simulink model "processor"  (R2024a)
settings: Solver=VariableStepAuto  StartTime=0.0  StopTime=10.0  RelTol=1e-3
libraries: simulink x10, hdlsllib x6
settings Model: Creator=alehay  LastModifiedBy=alehay

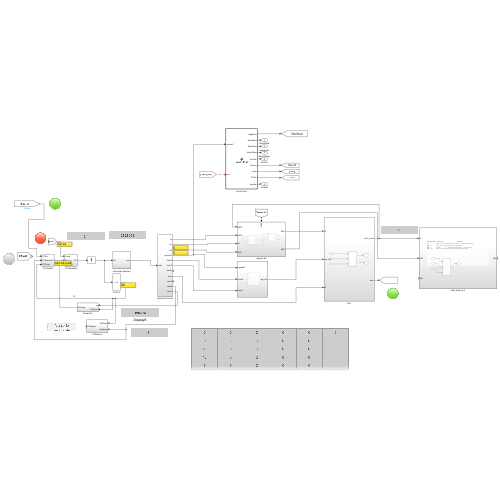
[thumbnail: Simulink's stored preview of the top-level diagram]
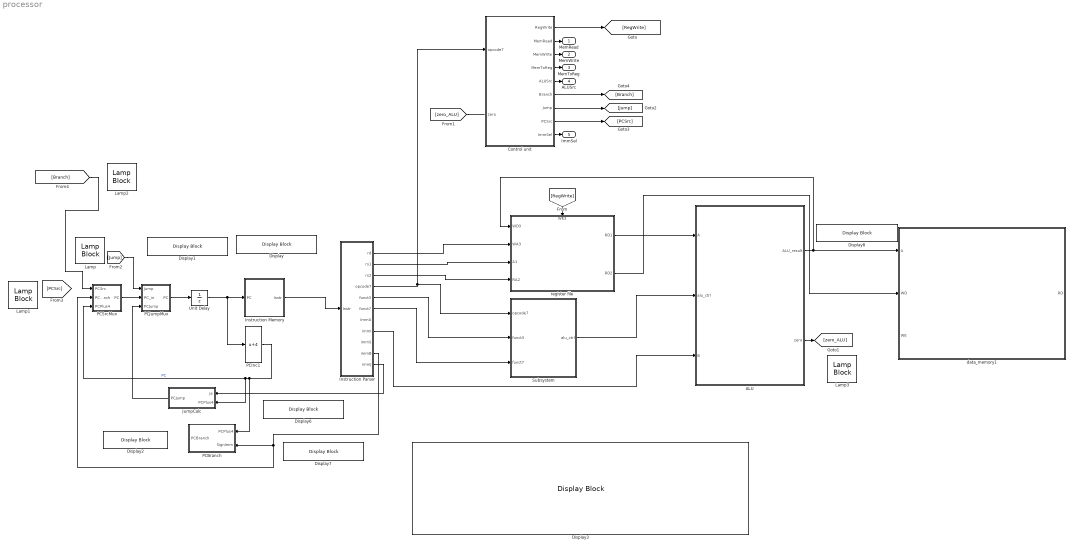
== system processor ==
  ALU : Subsystem
  Control unit : MATLAB Function  TreatAsAtomicUnit=on
  Display : DisplayBlock  LabelPosition=Hide  Format=Custom  Transparency=1  FormatString=%X
  Display{1,6..8} (4 alike) : DisplayBlock  LabelPosition=Hide  Transparency=1
  Display2 : DisplayBlock  LabelPosition=Hide  Format=long  Transparency=1
  Display3 : DisplayBlock  LabelPosition=Hide  Format=long  Transparency=1
  Instruction Memory : Subsystem
  Instruction Parser : Subsystem
  JumpCalc : Subsystem
  Lamp{,1..3} (4 alike) : LampBlock  LabelPosition=Hide
  PCBranch : Subsystem
  PCInc1 : Bias  Bias=4  SaturateOnIntegerOverflow=off
  PCJumpMux : Subsystem
  PCSrcMux : Subsystem
  Subsystem : Subsystem
  Unit Delay : UnitDelay  SampleTime=0.1  HasFrameUpgradeWarning=on
  data_memory1 : Subsystem
  register file : Subsystem
      settings: PortSchema="{\"entries\":[{\"content\":{\"sides\":[{\"content\":{\"connectorIds\":[\"In1\",\"In2\",\"In3\",\"In4\"]},\"type\":\"ConnectorPlacement.EquallySpacedRectSide\",\"uuid\":\"2ce0f731-262a-4c53-91f0-cda99c1614e4\"},{\"content\":{\"connectorIds\":[\"Out1\",\"Out2\"],\"side\":\"RIGHT\"},\"type\":\"ConnectorPlacement.EquallySpacedRectSide\",\"uuid\":\"7b2b7fe1-676c-4333-9af8-1b5ede950b35\"},{\"content\":{\"connectorIds\":[\"In5\"],\"side\":\"TOP\"},\"type\":\"ConnectorPlacement.EquallySpacedRectSide\",\"uuid\":\"79cd4f04-c8ad-45c4-b16c-19b290692dc4\"}]},\"type\":\"ConnectorPlacement.EquallySpacedConnector\",\"uuid\":\"48f070a2-9602-434c-b37d-35cc322e3ca0\"}],\"packageUris\":[\"http://schema.mathworks.com/mf0/Connector/R2020b\"],\"version\":\"1.0\"}"
  MemRead : Outport
  MemWrite : Outport  Port=2
  MemToReg : Outport  Port=3
  ALUSrc : Outport  Port=4
  ImmSel : Outport  Port=5
  wires:
  Control unit/5(ALUSrc) -> ALUSrc/1
  Instruction Parser/2(rs1) -> register file/3(A1)
  Control unit/9(ImmSel) -> ImmSel/1
  Control unit/3(MemWrite) -> MemWrite/1
  ALU/2(zero) -> [zero_ALU]
  Instruction Memory/1(Instr) -> Instruction Parser/1(Instr)
  Control unit/7(Jump) -> [Jump]
  register file/1(RD1) -> ALU/1(A)
  JumpCalc/1(PCJump) -> PCJumpMux/3(PCJump)
  register file/2(RD2) -> data_memory1/2(WD)
  Control unit/4(MemToReg) -> MemToReg/1
  Control unit/2(MemRead) -> MemRead/1
  Instruction Parser/6(funct7) -> Subsystem/3(funct7)
  Instruction Parser/4(opcode7) -> Control unit/1(opcode7), Subsystem/1(opcode7)
  [RegWrite] -> register file/5(WE3)
  Instruction Parser/5(funct3) -> Subsystem/2(funct3)
  PCInc1/1 -> PCSrcMux/3(PCPlus4), JumpCalc/2(PCPlus4), PCBranch/1(PCPlus4)  "PC"
  [zero_ALU] -> ?
  Control unit/1(RegWrite) -> [RegWrite]
  Instruction Parser/10(immB) -> PCSrcMux/2(PCBranch), PCBranch/2(SignImm)
  Instruction Parser/11(immJ) -> JumpCalc/1(ja)
  PCSrcMux/1(PC) -> PCJumpMux/2(PC_in)
  Control unit/8(PCSrc) -> [PCSrc]
  Unit Delay/1 -> Instruction Memory/1(PC), PCInc1/1
  Instruction Parser/3(rs2) -> register file/4(RA2)
  Control unit/6(Branch) -> [Branch]
  Instruction Parser/8(immI) -> ALU/3(B)
  Subsystem/1(alu_ctrl) -> ALU/2(alu_ctrl)
  [Jump] -> PCJumpMux/1(Jump)
  Instruction Parser/1(rd) -> register file/2(WA3)
  PCJumpMux/1(PC) -> Unit Delay/1
  ALU/1(ALU_result) -> data_memory1/1(A), register file/1(WD3)
  [Branch] -> PCSrcMux/1(PCSrc)

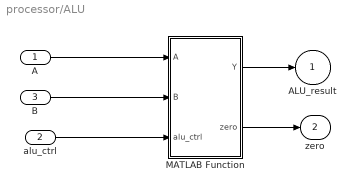
== system processor/ALU ==
  A : Inport
  alu_ctrl : Inport  Port=2
  B : Inport  Port=3
  MATLAB Function : MATLAB Function  TreatAsAtomicUnit=on
  ALU_result : Outport
  zero : Outport  Port=2
  wires:
  A/1 -> MATLAB Function/1(A)
  B/1 -> MATLAB Function/2(B)
  alu_ctrl/1 -> MATLAB Function/3(alu_ctrl)
  MATLAB Function/1(Y) -> ALU_result/1
  MATLAB Function/2(zero) -> zero/1

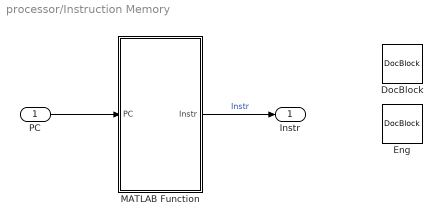
== system processor/Instruction Memory ==
  PC : Inport
  DocBlock : simulink/Model-Wide Utilities/DocBlock  DocumentType=Text
      content=|
      | Память команд имеет один порт чтения. На адресный вход A подается
      | 32-битный адрес команды, после чего на выходе RD появляется
      | 32-битное число (т.е. команда), прочитанное из памяти по этому адресу.
  Eng : simulink/Model-Wide Utilities/DocBlock  DocumentType=Text
      content=|
      | The instruction memory has a single read port.1 It takes a 32-bit
      | instruction address input, A, and reads the 32-bit data (i.e., instruction)
      | from that address onto the read data output, RD.
  MATLAB Function : MATLAB Function  TreatAsAtomicUnit=on
  Instr : Outport  OutDataTypeStr=fixdt(0,32,0)
  wires:
  PC/1 -> MATLAB Function/1(PC)
  MATLAB Function/1(Instr) -> Instr/1  "Instr"

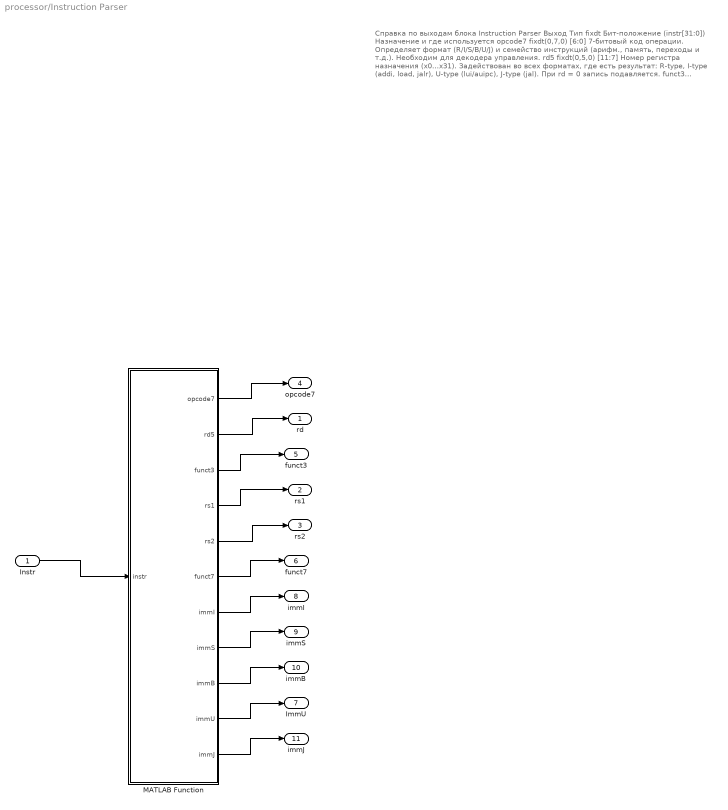
== system processor/Instruction Parser ==
  note: Справка по выходам блока Instruction Parser
      |
      | Выход
      | Тип fixdt
      | Бит-положение (instr[31:0])
      | Назначение и где используется
      |
      | opcode7
      | fixdt(0,7,0)
      | [6:0]
      | 7-битовый код операции. Определяет формат (R/I/S/B/U/J) и семейство инструкций (арифм., память, переходы и т.д.). Необходим для декодера управления.
      |
      | rd5
      | fixdt(0,5,0)
      | [11:7]
      | Номер регистра назначения (x0…x31). Задействован во всех форматах, где есть результат: R-type, I-type (addi, load, jalr), U-type (lui/auipc), J-type (jal). При rd = 0 запись подавляется.
      |
      | funct3
      | fixdt(0,3,0)
      | [14:12]
      | 3-битовое поле доп. кодировки операции. Совместно с opcode7 и/или funct7 окончательно выбирает инструкцию (например, add/sub, beq/bne/blt…).
      |
      | rs1
      | fixdt(0,5,0)
      | [19:15]
      | Номер первого исходного регистра. Используется во всех форматах, кроме U-type.
      |
      | rs2
      | fixdt(0,5,0)
      | [24:20]
      | Номер второго исходного регистра. Присутствует в R-type, S-type (store) и B-type (branch).
      |
      | funct7
      | fixdt(0,7,0)
      | [31:25]
      | 7-битовое поле расширенной функции. Отличает пары вроде add/sub, srl/sra, mul/div и др. Содержит 0x00, 0x20, 0x01 в базовом RV32IM.
      |
      | immI
      | fixdt(1,32,0)
      | sign-ext из [31:20]
      | 12-битное знаковое immed. для I-type (addi, lw, jalr, csrs …). Представляет диапазон −2048…+2047.
      |
      | immS
      | fixdt(1,32,0)
      | sign-ext из [31:25]+[11:7]
      | 12-битное знаковое immed. для S-type (store инструкции sw, sh, sb). Разделён на две части в коде.
      |
      | immB
      | fixdt(1,32,0)
      | sign-ext из [31], [7], [30:25], [11:8] затем <<1
      | 13-битное знаковое смещение для ветвлений B-type (beq, blt…). Младший бит всегда 0 — адрес выровнен по 2 байта. Диапазон ±4 кБ.
      |
      | immU
      | fixdt(1,32,0)
      | sign-ext из [31:12] затем <<12
      | 20-битное верхнее immediate для U-type (lui, auipc). Занимает старшие 20 бит результирующего слова, младшие 12 бит — нули.
      |
      | immJ
      | fixdt(1,32,0)
      | sign-ext из [31], [19:12], [20], [30:21]
      | 21-битное знаковое смещение для J-type (jal). Вычисляется с <<1; младший бит адреса всегда 0. Диапазон ±1 МБ.
  Instr : Inport
  MATLAB Function : MATLAB Function  TreatAsAtomicUnit=on
  rd : Outport
  rs1 : Outport  Port=2
  rs2 : Outport  Port=3
  opcode7 : Outport  Port=4
  funct3 : Outport  Port=5  OutDataTypeStr=fixdt(0,3,0)
  funct7 : Outport  Port=6  OutDataTypeStr=fixdt(0,7,0)
  ImmU : Outport  Port=7
  immI : Outport  Port=8
  immS : Outport  Port=9
  immB : Outport  Port=10
  immJ : Outport  Port=11
  wires:
  Instr/1 -> MATLAB Function/1(instr)
  MATLAB Function/1(opcode7) -> opcode7/1
  MATLAB Function/4(rs1) -> rs1/1
  MATLAB Function/3(funct3) -> funct3/1
  MATLAB Function/2(rd5) -> rd/1
  MATLAB Function/5(rs2) -> rs2/1
  MATLAB Function/6(funct7) -> funct7/1
  MATLAB Function/7(immI) -> immI/1
  MATLAB Function/8(immS) -> immS/1
  MATLAB Function/9(immB) -> immB/1
  MATLAB Function/10(immU) -> ImmU/1
  MATLAB Function/11(immJ) -> immJ/1

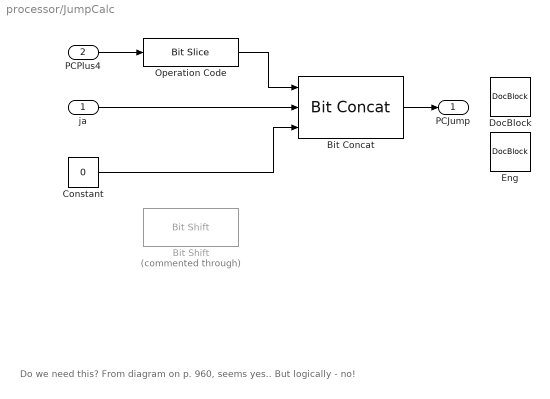
== system processor/JumpCalc ==
  note: Do we need this? From diagram on p. 960, seems yes.. But logically - no!
  ja : Inport
  PCPlus4 : Inport  Port=2
  Bit Concat : hdlsllib/Logic and Bit Operations/Bit Concat  numInputs=3
  Bit Shift : hdlsllib/Logic and Bit Operations/Bit Shift  Commented=through  mode=Shift Left Logical  N=2
  Constant : Constant  Value=0  OutDataTypeStr=fixdt(0,2,0)
  DocBlock : simulink/Model-Wide Utilities/DocBlock  DocumentType=Text
      content=|
      | Команда безусловного перехода j записывает новое значение в счетчик команд.
      | Два младших бита нового значения всегда равны нулю, потому что длина любой
      | команды равна четырем байтам, следовательно, ее адрес всегда кратен
      | четырем. Следующие 26 бит процессор возьмет из поля адреса перехода (jump
      | address field) Instr25:0. Четыре оставшихся старших бита будут равны четырем
      | старшим битам предыдущего значения счетчика команд.
  Eng : simulink/Model-Wide Utilities/DocBlock  DocumentType=Text
      content=|
      | The jump instruction, j, writes a new value into the PC. The two least significant
      | bits of the PC are always 0, because the PC is word aligned (i.e., always a multiple
      | of 4). The next 26 bits are taken from the jump address field in Instr25:0. The
      | upper four bits are taken from the old value of the PC.
  Operation Code : hdlsllib/Logic and Bit Operations/Bit Slice  lidx=31  ridx=28
  PCJump : Outport
  wires:
  Bit Concat/1 -> PCJump/1
  PCPlus4/1 -> Operation Code/1
  ja/1 -> Bit Concat/2
  Operation Code/1 -> Bit Concat/1
  Constant/1 -> Bit Concat/3

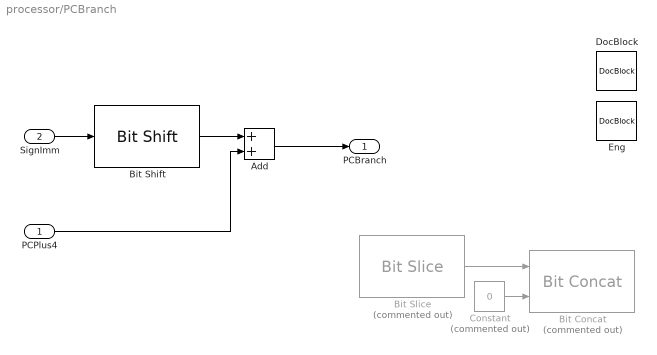
== system processor/PCBranch ==
  PCPlus4 : Inport
  SignImm : Inport  Port=2
  Add : Sum  OutDataTypeStr=fixdt(0,32,0)  AccumDataTypeStr=fixdt(0,32,0)
  Bit Concat : hdlsllib/Logic and Bit Operations/Bit Concat  Commented=on  numInputs=2
  Bit Shift : hdlsllib/Logic and Bit Operations/Bit Shift  mode=Shift Left Logical  N=2
  Bit Slice : hdlsllib/Logic and Bit Operations/Bit Slice  Commented=on  lidx=29  ridx=0
  Constant : Constant  Commented=on  Value=0  OutDataTypeStr=fixdt(0,2,0)
  DocBlock : simulink/Model-Wide Utilities/DocBlock  DocumentType=Text
      content=|
      | Смещение указывает, сколько команд нужно перепрыгнуть, прежде чем
      | продолжить выполнение программы. Таким образом, над значением
      | непосредственного операнда надо выполнить операцию знакового
      | расширения, поле чего умножить его на четыре, чтобы получить новое
      | значение счетчика команд: PC_in = PC + 4 + SignImm * 4.
      | Новое значение счетчика команд на случай выполненного
      | условного перехода (PCBranch) вычисляется путем сдвига SignImm
      | влево на два разряда и последующего сложения с PCPlus4.
  Eng : simulink/Model-Wide Utilities/DocBlock  DocumentType=Text
      content=|
      | The offset
      | indicates the number of instructions to branch past. Hence, the immediate
      | must be sign-extended and multiplied by 4 to get the new program counter
      | value: PC′ = PC + 4 + SignImm × 4.
      | The next PC value
      | for a taken branch, PCBranch, is computed by shifting SignImm left
      | by 2 bits, then adding it to PCPlus4.
  PCBranch : Outport
  wires:
  SignImm/1 -> Bit Shift/1
  PCPlus4/1 -> Add/2
  Bit Shift/1 -> Add/1
  Add/1 -> PCBranch/1
  Bit Slice/1 -> Bit Concat/1
  Constant/1 -> Bit Concat/2

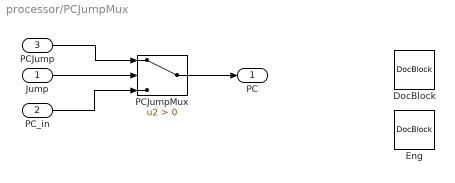
== system processor/PCJumpMux ==
  Jump : Inport
  PC_in : Inport  Port=2
  PCJump : Inport  Port=3
  DocBlock : simulink/Model-Wide Utilities/DocBlock  DocumentType=Text
      content=|
      | Команда безусловного перехода j записывает новое значение в счетчик команд.
      | Два младших бита нового значения всегда равны нулю, потому что длина любой
      | команды равна четырем байтам, следовательно, ее адрес всегда кратен
      | четырем. Следующие 26 бит процессор возьмет из поля адреса перехода (jump
      | address field) Instr25:0. Четыре оставшихся старших бита будут равны четырем
      | старшим битам предыдущего значения счетчика команд.
  Eng : simulink/Model-Wide Utilities/DocBlock  DocumentType=Text
      content=|
      | The jump instruction, j, writes a new value into the PC. The two least significant
      | bits of the PC are always 0, because the PC is word aligned (i.e., always a multiple
      | of 4). The next 26 bits are taken from the jump address field in Instr25:0. The
      | upper four bits are taken from the old value of the PC.
  PCJumpMux : Switch  Criteria=u2 > Threshold  SaturateOnIntegerOverflow=off  InputSameDT=off
  PC : Outport
  wires:
  PCJumpMux/1 -> PC/1
  Jump/1 -> PCJumpMux/2
  PCJump/1 -> PCJumpMux/1
  PC_in/1 -> PCJumpMux/3

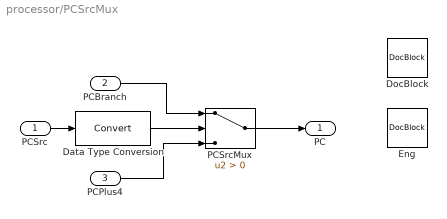
== system processor/PCSrcMux ==
  PCSrc : Inport  OutDataTypeStr=boolean
  PCBranch : Inport  Port=2
  PCPlus4 : Inport  Port=3
  Data Type Conversion : DataTypeConversion  SaturateOnIntegerOverflow=off  RndMeth=Floor
  DocBlock : simulink/Model-Wide Utilities/DocBlock  DocumentType=Text
      content=|
      | Мультиплексор, чтобы выбрать, какое именно
      | значение присвоить PC_in – PCPlus4 или PCBranch. PCBranch
      | используется тогда, когда выполняется команда условного перехода и
      | установлен флаг нуля.
  Eng : simulink/Model-Wide Utilities/DocBlock  DocumentType=Text
      content=|
      | The multiplexer to choose PC′ from either
      | PCPlus4 or PCBranch. PCBranch is selected if the instruction is a branch
      | and the Zero flag is asserted.
  PCSrcMux : Switch  Criteria=u2 > Threshold  SaturateOnIntegerOverflow=off  InputSameDT=off
  PC : Outport
  wires:
  PCSrc/1 -> Data Type Conversion/1
  PCPlus4/1 -> PCSrcMux/3
  PCSrcMux/1 -> PC/1
  PCBranch/1 -> PCSrcMux/1
  Data Type Conversion/1 -> PCSrcMux/2

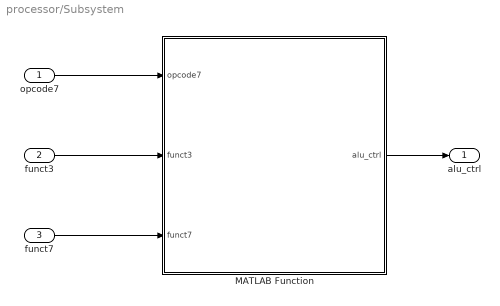
== system processor/Subsystem ==
  opcode7 : Inport
  funct3 : Inport  Port=2
  funct7 : Inport  Port=3
  MATLAB Function : MATLAB Function  TreatAsAtomicUnit=on
  alu_ctrl : Outport
  wires:
  opcode7/1 -> MATLAB Function/1(opcode7)
  funct3/1 -> MATLAB Function/2(funct3)
  funct7/1 -> MATLAB Function/3(funct7)
  MATLAB Function/1(alu_ctrl) -> alu_ctrl/1

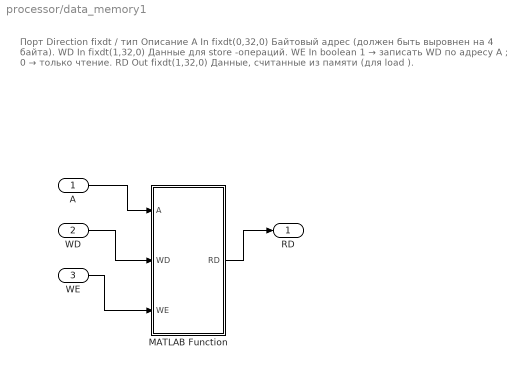
== system processor/data_memory1 ==
  note: Порт
      | Direction
      | fixdt / тип
      | Описание
      |
      | A
      | In
      | fixdt(0,32,0)
      | Байтовый адрес (должен быть выровнен на 4 байта).
      |
      | WD
      | In
      | fixdt(1,32,0)
      | Данные для store -операций.
      |
      | WE
      | In
      | boolean
      | 1 → записать WD по адресу A ; 0 → только чтение.
      |
      | RD
      | Out
      | fixdt(1,32,0)
      | Данные, считанные из памяти (для load ).
  A : Inport
  WD : Inport  Port=2
  WE : Inport  Port=3
  MATLAB Function : MATLAB Function  TreatAsAtomicUnit=on
  RD : Outport
  wires:
  MATLAB Function/1(RD) -> RD/1
  A/1 -> MATLAB Function/1(A)
  WD/1 -> MATLAB Function/2(WD)
  WE/1 -> MATLAB Function/3(WE)

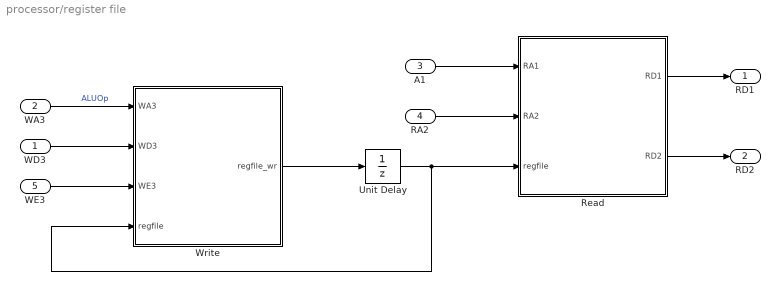
== system processor/register file ==
  WD3 : Inport
  WA3 : Inport  Port=2
  A1 : Inport  Port=3
  RA2 : Inport  Port=4
  WE3 : Inport  Port=5  OutDataTypeStr=boolean
  Read : MATLAB Function  TreatAsAtomicUnit=on
  Unit Delay : UnitDelay  SampleTime=-1  HasFrameUpgradeWarning=on
  Write : MATLAB Function  TreatAsAtomicUnit=on
  RD1 : Outport  OutDataTypeStr=fixdt(0,32,0)
  RD2 : Outport  Port=2  OutDataTypeStr=fixdt(0,32,0)
  wires:
  A1/1 -> Read/1(RA1)
  RA2/1 -> Read/2(RA2)
  Read/2(RD2) -> RD2/1
  WA3/1 -> Write/1(WA3)  "ALUOp"
  Read/1(RD1) -> RD1/1
  WD3/1 -> Write/2(WD3)
  WE3/1 -> Write/3(WE3)
  Write/1(regfile_wr) -> Unit Delay/1
  Unit Delay/1 -> Write/4(regfile), Read/3(regfile)

== matlab function processor/data_memory1/MATLAB Function ==
  data: A input fixdt(0,32,0) size=[1 1]; RD output fixdt(0,32,0) size=[1 1]; WD input fixdt(0,32,0) size=[1 1]; WE input boolean size=[1 1]
% === Data-Memory RV32I (byte-addr., 32-bit words) ===
%  *входы*   A  : fi, fixdt(0,32,0)  — байтовый адрес  
%            WD : fi, fixdt(0,32,0)  — данные для записи  
%            WE : logical            — разрешение записи (1 = store)  
%  *выходы*  RD : fi, fixdt(1,32,0)  — данные чтения (load)  
%
%   • чтение асинхронное: RD меняется сразу при изменении A;  
%   • запись синхронная по «такту вызова» функции: если WE=1, новое
%     значение станет видимым при следующем вызове (поведение “write-after-read”).

function RD = fcn(A, WD, WE)   %#codegen
    persistent mem
    if isempty(mem)
        mem = zeros(1024,1,'uint32');   % 4 КБ = 1024 слов × 4 байта
    end

    addr     = uint32(A);              % fi → беззн. 32-бит
    word_idx = bitshift(addr, -2);     % адрес слова (addr / 4)

    in_range = word_idx < 1024;        % защита от выхода за пределы

    % ---- запись --------------------------------------------------------
    if WE && in_range
        mem(double(word_idx) + 1) = uint32(WD);
    end

    % ---- чтение --------------------------------------------------------
    if in_range
        RD_u = mem(double(word_idx) + 1);
    else
        RD_u = uint32(0);
    end

    RD = fi(int32(RD_u), 0, 32, 0);    % SFix_32_0 на выход
end

== matlab function processor/register file/Read ==
  data: RA1 input fixdt(0,5,0) size=[1 1]; RD1 output fixdt(0,32,0) size=[1 1]; RA2 input fixdt(0,5,0) size=[1 1]; RD2 output fixdt(0,32,0) size=[1 1]; regfile input fixdt(0,32,0) size=[32]
function [RD1, RD2] = fcn(RA1, RA2, regfile) %#codegen
% RA1, RA2 : fi, fixdt(0,5,0)
% regfile  : fi(0,32,0) [32×1]
% RD1, RD2 : fi(0,32,0)

    %------ жёстко объявляем выходы того же типа ------
    RD1 = fi(0, 0, 32, 0);
    RD2 = fi(0, 0, 32, 0);
    %--------------------------------------------------

    a1 = uint8(RA1);
    a2 = uint8(RA2);

    RD1(:) = regfile(int32(a1)+1);
    RD2(:) = regfile(int32(a2)+1);

    if a1 == 0      % x0 всегда 0
        RD1(:) = 0; % можно и просто 0 — константа
    end
    if a2 == 0
        RD2(:) = 0;
    end
end

== matlab function processor/Instruction Parser/MATLAB Function ==
  data: instr input fixdt(0,32,0) size=[1 1]; opcode7 output fixdt(0,7,0) size=[1 1]; rd5 output; funct3 output; rs1 output; rs2 output; funct7 output; immI output; immS output; immB output; immU output; immJ output
function [opcode7, rd5, funct3, rs1, rs2, funct7, ...
          immI, immS, immB, immU, immJ] = InstructionParser(instr)
%#codegen

u = uint32(instr);

%------------- 1. Статические поля ----------------------------------------
opcode7 = fi(bitand(u, 127)             , 0, 7, 0);        % [6:0]
rd5     = fi(bitand(bitshift(u,-7),31)  , 0, 5, 0);        % [11:7]
funct3  = fi(bitand(bitshift(u,-12),7)  , 0, 3, 0);        % [14:12]
rs1     = fi(bitand(bitshift(u,-15),31) , 0, 5, 0);        % [19:15]
rs2     = fi(bitand(bitshift(u,-20),31) , 0, 5, 0);        % [24:20]
funct7  = fi(bitand(bitshift(u,-25),127), 0, 7, 0);        % [31:25]

%------------- 2. Знаковое расширение N-битного поля ----------------------
extend = @(raw,N) int32( ...
            bitshift(bitshift(int32(raw), 32-N), -(32-N)));

%------------- 3. I-type --------------------------------------------------
immI = fi( extend(bitshift(u,-20),12) , 1, 32, 0);

%------------- 4. S-type --------------------------------------------------
tmpS = bitor(bitshift(bitand(u,hex2dec('FE000000')),-25), ... % [11:5]
             bitand(bitshift(u,-7),31));                       % [4:0]
immS = fi( extend(tmpS,12)                , 1, 32, 0);

%------------- 5. B-type (смещение уже кратно 2) --------------------------
tmpB = bitor( bitshift(bitand(u,hex2dec('80000000')),-19), ... 
       bitor( bitshift(bitand(u,hex2dec('7E000000')),-20), ... 
       bitor( bitshift(bitand(u,hex2dec('00000F00')),-7) , ... 
               bitshift(bitand(u,hex2dec('00000080')), 4))));   
immB = fi( extend(tmpB,13)                 , 1, 32, 0);

%------------- 6. U-type (<<12) -------------------------------------------
tmpU = bitshift(u,-12);                    % imm[31:12]
immU = fi( extend(tmpU,20), 0, 32, 0);     % знак не нужен
immU = bitshift(immU,12);                  % <<12

%------------- 7. J-type (смещение кратно 2) ------------------------------
tmpJ = bitor( bitshift(bitand(u,hex2dec('80000000')),-11), ... % imm[20]
       bitor( bitshift(bitand(u,hex2dec('7FE00000')),-20), ... % imm[10:1]
       bitor( bitshift(bitand(u,hex2dec('00100000')),-9) , ... % imm[11]
               bitand(u,hex2dec('000FF000')))));               % imm[19:12]
immJ = fi( extend(tmpJ,21)                 , 1, 32, 0);
end

== matlab function processor/register file/Write ==
  data: WA3 input fixdt(0,5,0) size=[1 1]; WD3 input fixdt(0,32,0) size=[1 1]; WE3 input boolean size=[1 1]; regfile input fixdt(0,32,0) size=[32]; regfile_wr output size=[32]
% === Блок записи регистров RISC-V (WA3 - fixdt(0,5,0)) ===
function regfile_wr = fcn(WA3, WD3, WE3, regfile) %#codegen
    % фиксированный вектор 32×1
    regfile_wr = uint32(zeros(32,1));

    % перенос прошлого состояния (если пришёл другой размер)
    n = min(numel(regfile),32);
    regfile_wr(1:n) = regfile(1:n);

    wa = uint8(WA3);
    if WE3 && wa~=0
        regfile_wr(int32(wa)+1) = WD3;
    end
    regfile_wr(1) = uint32(0);   % x0 всегда 0
end

== matlab function processor/Subsystem/MATLAB Function ==
  data: opcode7 input fixdt(0,7,0) size=[1 1]; alu_ctrl output fixdt(0,4,0) size=[1 1]; funct3 input fixdt(0,3,0) size=[1 1]; funct7 input fixdt(0,7,0) size=[1 1]
% === ALU Control для RV32I (coder-safe) ===
function alu_ctrl = fcn(opcode7, funct3, funct7) %#codegen
% Входы:
%   opcode7 : fi, fixdt(0,7,0)  – instr[6:0]
%   funct3  : fi, fixdt(0,3,0)  – instr[14:12]
%   funct7  : fi, fixdt(0,7,0)  – instr[31:25]
% Выход:
%   alu_ctrl: fi, fixdt(0,4,0)  – код ALU:
%             0 ADD  1 SUB  2 AND  3 OR  4 XOR
%             5 SLL  6 SRL  7 SRA  8 SLT 9 SLTU

% --- приведение входов к uint8 ------------------------------------------
op = uint8(opcode7);
f3 = uint8(funct3);
f7 = uint8(funct7);

ctrl = uint8(0);     % по умолчанию ADD

% --- декодирование ------------------------------------------------------
switch op
    case uint8(hex2dec('33'))      % R-type
        switch f3
            case 0   % ADD / SUB
                if f7 == uint8(32)
                    ctrl = uint8(1);     % SUB
                else
                    ctrl = uint8(0);     % ADD
                end
            case 1,  ctrl = uint8(5);    % SLL
            case 2,  ctrl = uint8(8);    % SLT
            case 3,  ctrl = uint8(9);    % SLTU
            case 4,  ctrl = uint8(4);    % XOR
            case 5                    % SRL / SRA
                if f7 == uint8(32)
                    ctrl = uint8(7);     % SRA
                else
                    ctrl = uint8(6);     % SRL
                end
            case 6,  ctrl = uint8(3);    % OR
            case 7,  ctrl = uint8(2);    % AND
        end

    case uint8(hex2dec('13'))      % I-type (имм.)
        switch f3
            case 0,  ctrl = uint8(0);    % ADDI
            case 2,  ctrl = uint8(8);    % SLTI
            case 3,  ctrl = uint8(9);    % SLTIU
            case 4,  ctrl = uint8(4);    % XORI
            case 6,  ctrl = uint8(3);    % ORI
            case 7,  ctrl = uint8(2);    % ANDI
            case 1,  ctrl = uint8(5);    % SLLI
            case 5                    % SRLI / SRAI
                if f7 == uint8(32)
                    ctrl = uint8(7);     % SRAI
                else
                    ctrl = uint8(6);     % SRLI
                end
        end

    case { uint8(hex2dec('03')), ... % LOAD
           uint8(hex2dec('23')), ... % STORE
           uint8(hex2dec('67')), ... % JALR
           uint8(hex2dec('6F')), ... % JAL
           uint8(hex2dec('17')), ... % AUIPC
           uint8(hex2dec('37')) }    % LUI
        ctrl = uint8(0);             % всегда ADD

    case uint8(hex2dec('63'))        % BRANCH
        ctrl = uint8(1);             % SUB (для сравнения)
end

% --- возврат как fi ------------------------------------------------------
alu_ctrl = fi(ctrl, 0, 4, 0);
end

== matlab function processor/ALU/MATLAB Function ==
  data: A input fixdt(0,32,0) size=[1 1]; Y output fixdt(0,32,0) size=[1 1]; B input fixdt(1,32,0) size=[1 1]; alu_ctrl input fixdt(0,4,0) size=[1 1]; zero output boolean size=[1 1]
function [Y, zero] = fcn(A, B, alu_ctrl)   %#codegen
% A,B      : fi, fixdt(1,32,0)
% alu_ctrl : fi, fixdt(0,4,0)
% Y        : fi, fixdt(0,32,0)
% zero     : logical

% ---------- Жёстко объявляем выходы ----------
Y    = fi(0, 0, 32, 0);     % 1×1, unsigned, WL=32, FL=0
zero = false;               % logical скаляр
% ---------------------------------------------

a_s  = int32(A);             b_s  = int32(B);
a_u  = uint32(A);            b_u  = uint32(B);
sa   = bitand(b_u, 31);      % shift amount 0…31
ctrl = uint8(alu_ctrl);

switch ctrl
    case 0      % ADD
        Y(:) = fi(a_s + b_s, 0, 32, 0);

    case 1      % SUB
        Y(:) = fi(a_s - b_s, 0, 32, 0);

    case 2      % AND
        Y(:) = fi(bitand(a_u, b_u), 0, 32, 0);

    case 3      % OR
        Y(:) = fi(bitor(a_u, b_u), 0, 32, 0);

    case 4      % XOR
        Y(:) = fi(bitxor(a_u, b_u), 0, 32, 0);

    case 5      % SLL
        Y(:) = fi(bitshift(a_u,  sa), 0, 32, 0);

    case 6      % SRL
        Y(:) = fi(bitshift(a_u, -sa), 0, 32, 0);

    case 7      % SRA
        Y(:) = fi(bitshift(a_s, -sa), 0, 32, 0);

    case 8      % SLT
        Y(:) = fi(int32(a_s < b_s), 0, 32, 0);

    case 9      % SLTU
        Y(:) = fi(int32(a_u < b_u), 0, 32, 0);

    otherwise   % резерв
        Y(:) = fi(0, 0, 32, 0);
end

zero = (Y == 0);             % теперь Y уже гарантированно скаляр
end

== matlab function processor/Instruction Memory/MATLAB Function ==
  data: PC input fixdt(0,32,0) size=[1 1]; Instr output size=[1 1]
function Instr = fcn_rv(PC) %#codegen
% 64-word ROM with a small RV32I test program
persistent ROM
if isempty(ROM)
    ROM = fi(zeros(64,1), 0, 32, 0);   % 64 × 32-bit

    % addr    machine   assembly
%{
    ROM(1)  = hex2dec('00500113'); % addi x2,x0,5
    ROM(2)  = hex2dec('00C00193'); % addi x3,x0,12
    ROM(3)  = hex2dec('FF718393'); % addi x7,x3,-9
    ROM(4)  = hex2dec('0023E233'); % or   x4,x7,x2
    ROM(5)  = hex2dec('0041F2B3'); % and  x5,x3,x4
    ROM(6)  = hex2dec('004282B3'); % add  x5,x5,x4
    ROM(7)  = hex2dec('02728663'); % beq  x5,x7, end
    ROM(8)  = hex2dec('0041A233'); % slt  x4,x3,x4
    ROM(9)  = hex2dec('00020463'); % beq  x4,x0, around
    ROM(10) = hex2dec('00000293'); % addi x5,x0,0
    % --- around (0x0028) ---
    ROM(11) = hex2dec('0023A233'); % slt  x4,x7,x2
    ROM(12) = hex2dec('402383B3'); % sub  x7,x7,x2
    ROM(13) = hex2dec('0471A223'); % sw   x7,68(x3)
    ROM(14) = hex2dec('05002103'); % lw   x2,80(x0)
    ROM(15) = hex2dec('0080006F'); % jal  x0, end (+8)
    ROM(16) = hex2dec('00100113'); % (не исполнится)
    % --- end (0x0044) ---
    ROM(17) = hex2dec('04202A23'); % sw   x2,84(x0)
    ROM(18) = hex2dec('FFDFF06F'); % jal  x0, end (-4, «halt»)
%}

ROM(1)  = hex2dec('00001101');   % addi   sp, sp, -32
ROM(2)  = hex2dec('0000ce06');   % sw     ra, 28(sp)
ROM(3)  = hex2dec('0000cc22');   % sw     s0, 24(sp)
ROM(4)  = hex2dec('00001000');   % addi   s0, sp, 32
ROM(5)  = hex2dec('02100793');   % li     a5, 33
ROM(6)  = hex2dec('fef42623');   % sw     a5, -20(s0)
ROM(7)  = hex2dec('04d00793');   % li     a5, 77
ROM(8)  = hex2dec('fef42423');   % sw     a5, -24(s0)
ROM(9)  = hex2dec('fe042223');   % sw     zero, -28(s0)
ROM(10) = hex2dec('fec42703');   % lw     a4, -20(s0)
ROM(11) = hex2dec('fe842783');   % lw     a5, -24(s0)
ROM(12) = hex2dec('00e7db63');   % bge    a5, a4, 3a <.L2>
ROM(13) = hex2dec('fec42703');   % lw     a4, -20(s0)
ROM(14) = hex2dec('fe842783');   % lw     a5, -24(s0)
ROM(15) = hex2dec('40f707b3');   % sub    a5, a4, a5
ROM(16) = hex2dec('fef42223');   % sw     a5, -28(s0)
ROM(17) = hex2dec('0000a801');   % j      48 <.L4>
ROM(18) = hex2dec('fec42703');   % lw     a4, -20(s0)
ROM(19) = hex2dec('fe842783');   % lw     a5, -24(s0)
ROM(20) = hex2dec('000097ba');   % add    a5, a5, a4
ROM(21) = hex2dec('fef42223');   % sw     a5, -28(s0)
ROM(22) = hex2dec('00000001');   % nop
ROM(23) = hex2dec('000040f2');   % lw     ra, 28(sp)
ROM(24) = hex2dec('00004462');   % lw     s0, 24(sp)
ROM(25) = hex2dec('00006105');   % addi   sp, sp, 32
ROM(26) = hex2dec('00008082');   % ret

end

%------------------------------------------------------------------
% 1) делим PC на 4 (logical right shift на 2 бита)
% 2) переводим в double и +1 для 1-based
% 3) насыщаем, если вышли за пределы ПЗУ
%------------------------------------------------------------------
idx = bitshift(uint32(PC),-2);   % /4
idx = double(idx) + 1;           % 1-based
idx = min(idx, numel(ROM));      % saturation

Instr = ROM(idx);                % читаем слово из ПЗУ
end

== matlab function processor/Control unit ==
  data: opcode7 input fixdt(0,7,0); RegWrite output boolean size=[1 1]; MemRead output; MemWrite output; MemToReg output; ALUSrc output; Branch output; Jump output boolean size=[1 1]; PCSrc output boolean size=[1 1]; ImmSel output; zero input
function [RegWrite, MemRead, MemWrite, MemToReg, ...
          ALUSrc, Branch, Jump, PCSrc, ImmSel] = ControlUnit(opcode7, zero) %#codegen
%--------------------------------------------------------------------------
%  RV32I Control-Unit (однотактный вариант, без структур).
%
%  Входы
%     opcode7 : fi, fixdt(0,7,0)  – instr[6:0]  (выход InstructionParser)
%     zero    : logical           – флаг "результат-ноль" от ALU
%
%  Выходы (9 отдельных линий, фиксированные типы)
%     RegWrite, MemRead, MemWrite, MemToReg,
%     ALUSrc, Branch, Jump, PCSrc : logical
%     ImmSel : fi, fixdt(0,3,0)   (0=I, 1=S, 2=B, 3=U, 4=J)
%--------------------------------------------------------------------------

%--- значения «по-умолчанию» (NOP) ----------------------------------------
RegWrite = false;
MemRead  = false;
MemWrite = false;
MemToReg = false;
ALUSrc   = false;
Branch   = false;
Jump     = false;
PCSrc    = false;
ImmSel   = fi(0, 0, 3, 0);      % 3-битное беззнаковое

op = uint8(opcode7);            % удобно для switch

switch op
%===================== U-type =============================================
case uint8(hex2dec('37'))           % LUI
    RegWrite = true;
    ALUSrc   = true;
    ImmSel   = fi(3, 0, 3, 0);

case uint8(hex2dec('17'))           % AUIPC
    RegWrite = true;
    ALUSrc   = true;                % PC + imm (делает ALU)
    ImmSel   = fi(3, 0, 3, 0);

%===================== J-type =============================================
case uint8(hex2dec('6F'))           % JAL
    RegWrite = true;
    Jump     = true;
    PCSrc    = true;                % PC <- PC + imm
    ImmSel   = fi(4, 0, 3, 0);

case uint8(hex2dec('67'))           % JALR
    RegWrite = true;
    Jump     = true;
    ALUSrc   = true;                % rs1 + imm
    PCSrc    = true;
    ImmSel   = fi(0, 0, 3, 0);      % I-imm

%===================== Branch (B-type) ====================================
case uint8(hex2dec('63'))           % BEQ/BNE/BGE/BLT/…
    Branch   = true;
    PCSrc    = (zero ~= 0);         % ← всегда logical
    ImmSel   = fi(2, 0, 3, 0);      % B-imm
%===================== Load ===============================================
case uint8(hex2dec('03'))           % LB/LH/LW/…
    RegWrite = true;
    MemRead  = true;
    MemToReg = true;
    ALUSrc   = true;
    ImmSel   = fi(0, 0, 3, 0);      % I-imm

%===================== Store ==============================================
case uint8(hex2dec('23'))           % SB/SH/SW
    MemWrite = true;
    ALUSrc   = true;
    ImmSel   = fi(1, 0, 3, 0);      % S-imm

%===================== I-type ALU =========================================
case uint8(hex2dec('13'))           % ADDI/ANDI/ORI/…
    RegWrite = true;
    ALUSrc   = true;
    ImmSel   = fi(0, 0, 3, 0);      % I-imm

%===================== R-type ALU =========================================
case uint8(hex2dec('33'))           % ADD/SUB/AND/…
    RegWrite = true;
    % ALUSrc остаётся 0 (rs2)

otherwise                            % SYSTEM/FENCE/ECALL/NOP …
    % всё уже обнулено
end
end
